simulink model "model1"  (R2020a)
settings: Solver=FixedStepAuto  StartTime=0.0  StopTime=30  FixedStep=0.005  RelTol=1e-3
values from neighbouring files (symbols this model uses):
  g = 9.81    [fast_init.m]
  I1 = 1    [fast_init.m]
  I2 = 10    [fast_init.m]
  ini_theta1 = 0    [fast_init.m]
  ini_theta1_d = 0    [fast_init.m]
  ini_theta2 = 0    [fast_init.m]
  ini_theta2_d = 0    [fast_init.m]
  ini_w = 1    [fast_init.m]
  ini_w_d = 0    [fast_init.m]
  ini_x0 = 0    [fast_init.m]
  ini_x0_d = 0    [fast_init.m]
  ini_x1 = ini_x0+r1*cos(pi/2 - ini_theta1)    [fast_init.m]
  ini_x1_d = 0    [fast_init.m]
  ini_x2 = ini_xH + r2*cos(pi/2 - ini_theta2)    [fast_init.m]
  ini_x2_d = 0    [fast_init.m]
  ini_y0 = 0.4    [fast_init.m]
  ini_y0_d = 0    [fast_init.m]
  ini_y1 = ini_y0+r1*sin(pi/2 - ini_theta1)    [fast_init.m]
  ini_y1_d = 0    [fast_init.m]
  ini_y2 = ini_yH + r2*sin(pi/2 - ini_theta2)    [fast_init.m]
  ini_y2_d = 0    [fast_init.m]
  M1 = 1    [fast_init.m]
  M2 = 10    [fast_init.m]
  r1 = 0.5    [fast_init.m]
  r2 = 0.4    [fast_init.m]
  theta1_des = 0    [fast_init.m]
libraries: cstblocks x6, simulink x1
settings Model: Creator=fabia  LastModifiedBy=mic-ciciolla

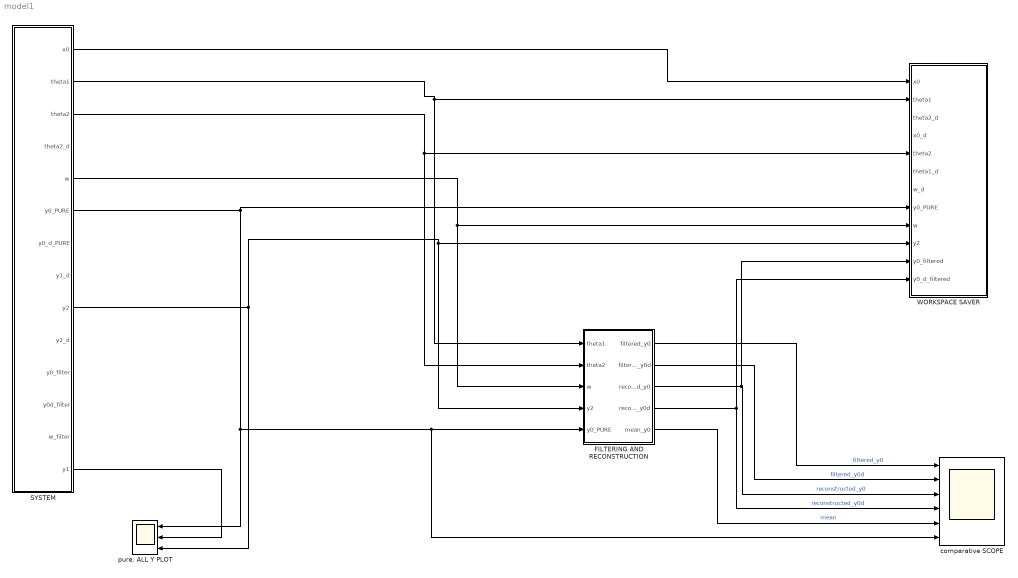
== system model1 ==
  FILTERING AND RECONSTRUCTION : Subsystem
  SYSTEM : Subsystem
  WORKSPACE SAVER : Subsystem
  comparative SCOPE : Scope  NumInputPorts=6
  pure: ALL Y PLOT : Scope  NumInputPorts=3
  wires:
  SYSTEM/6(y0_PURE) -> WORKSPACE SAVER/8(y0_PURE), pure: ALL Y PLOT/1, FILTERING AND RECONSTRUCTION/5(y0_PURE), comparative SCOPE/6
  SYSTEM/9(y2) -> FILTERING AND RECONSTRUCTION/4(y2), WORKSPACE SAVER/10(y2), pure: ALL Y PLOT/3
  SYSTEM/1(x0) -> WORKSPACE SAVER/1(x0)
  SYSTEM/2(theta1) -> FILTERING AND RECONSTRUCTION/1(theta1), WORKSPACE SAVER/2(theta1)
  SYSTEM/3(theta2) -> FILTERING AND RECONSTRUCTION/2(theta2), WORKSPACE SAVER/5(theta2)
  SYSTEM/5(w) -> FILTERING AND RECONSTRUCTION/3(w), WORKSPACE SAVER/9(w)
  SYSTEM/14(y1) -> pure: ALL Y PLOT/2
  FILTERING AND RECONSTRUCTION/1(filtered_y0) -> comparative SCOPE/1  "filtered_y0"
  FILTERING AND RECONSTRUCTION/2(filtered_y0d) -> comparative SCOPE/2  "filtered_y0d"
  FILTERING AND RECONSTRUCTION/4(reconstructed_y0d) -> WORKSPACE SAVER/12(y0_d_filtered), comparative SCOPE/4  "reconstructed_y0d"
  FILTERING AND RECONSTRUCTION/3(reconstructed_y0) -> WORKSPACE SAVER/11(y0_filtered), comparative SCOPE/3  "reconstructed_y0"
  FILTERING AND RECONSTRUCTION/5(mean_y0) -> comparative SCOPE/5  "mean"

== system model1/FILTERING AND RECONSTRUCTION ==
  theta1 : Inport
  theta2 : Inport  Port=2
  w : Inport  Port=3
  y2 : Inport  Port=4
  y0_PURE : Inport  Port=5
  FILTERING BLOCK : Subsystem
  RECONSTRUCTION BLOCK : Subsystem
  comparative SCOPE : Scope  NumInputPorts=5
  mean : MATLAB Function  TreatAsAtomicUnit=on
  filtered_y0 : Outport
  filtered_y0d : Outport  Port=2
  reconstructed_y0 : Outport  Port=3
  reconstructed_y0d : Outport  Port=4
  mean_y0 : Outport  Port=5
  wires:
  theta1/1 -> RECONSTRUCTION BLOCK/1(theta1)
  y0_PURE/1 -> FILTERING BLOCK/1(y0_PURE), comparative SCOPE/1
  y2/1 -> RECONSTRUCTION BLOCK/4(y2)
  theta2/1 -> RECONSTRUCTION BLOCK/2(theta2)
  RECONSTRUCTION BLOCK/1(reconstruct_y0) -> comparative SCOPE/2, mean/1(recon), reconstructed_y0/1
  FILTERING BLOCK/2(y0_d) -> filtered_y0d/1, comparative SCOPE/5  "filtered_y0d"
  RECONSTRUCTION BLOCK/2(recontruct_y0d) -> comparative SCOPE/3, reconstructed_y0d/1
  w/1 -> RECONSTRUCTION BLOCK/3(w)
  FILTERING BLOCK/1(y0) -> mean/2(filtered), filtered_y0/1, comparative SCOPE/4  "filtered_y0"
  mean/1(y) -> mean_y0/1

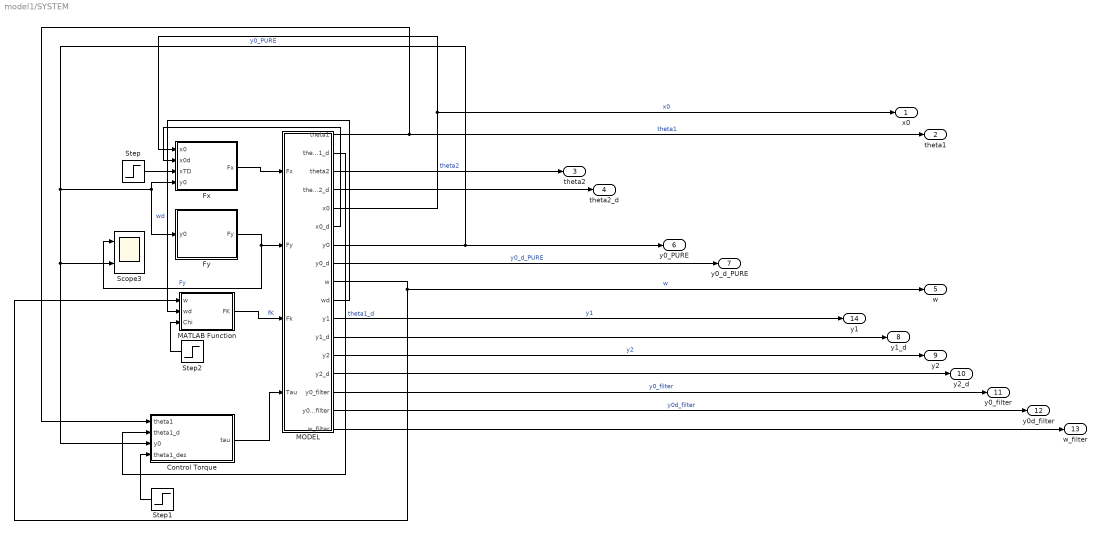
== system model1/SYSTEM ==
  Control Torque : MATLAB Function  TreatAsAtomicUnit=on
  Fx : MATLAB Function  TreatAsAtomicUnit=on
  Fy : MATLAB Function  TreatAsAtomicUnit=on
  MATLAB Function : MATLAB Function  TreatAsAtomicUnit=on
  MODEL : Subsystem
  Scope3 : Scope  NumInputPorts=2
  Step : Step  Time=0  After=0  SampleTime=0
  Step1 : Step  Time=0  After=theta1_des  SampleTime=0
  Step2 : Step  Time=0  After=0.0  SampleTime=0
  x0 : Outport
  theta1 : Outport  Port=2
  theta2 : Outport  Port=3
  theta2_d : Outport  Port=4
  w : Outport  Port=5
  y0_PURE : Outport  Port=6
  y0_d_PURE : Outport  Port=7
  y1_d : Outport  Port=8
  y2 : Outport  Port=9
  y2_d : Outport  Port=10
  y0_filter : Outport  Port=11
  y0d_filter : Outport  Port=12
  w_filter : Outport  Port=13
  y1 : Outport  Port=14
  wires:
  MODEL/2(theta1_d) -> Control Torque/2(theta1_d)  "theta1_d"
  MATLAB Function/1(FK) -> MODEL/3(Fk)  "fK"
  MODEL/9(w) -> w/1, MATLAB Function/1(w)  "w"
  MODEL/11(y1) -> y1/1  "y1"
  MODEL/14(y2_d) -> y2_d/1
  Fy/1(Fy) -> Scope3/1, MODEL/2(Fy)  "Fy"
  MODEL/17(w_filter) -> w_filter/1
  MODEL/12(y1_d) -> y1_d/1
  MODEL/5(x0) -> x0/1, Fx/1(x0)  "x0"
  MODEL/13(y2) -> y2/1  "y2"
  Fx/1(Fx) -> MODEL/1(Fx)
  MODEL/7(y0) -> y0_PURE/1, Control Torque/3(y0), Scope3/2, Fx/4(y0), Fy/1(y0)  "y0_PURE"
  MODEL/8(y0_d) -> y0_d_PURE/1  "y0_d_PURE"
  MODEL/1(theta1) -> Control Torque/1(theta1), theta1/1  "theta1"
  MODEL/15(y0_filter) -> y0_filter/1  "y0_filter"
  MODEL/3(theta2) -> theta2/1  "theta2"
  Step/1 -> Fx/3(xTD)
  MODEL/4(theta2_d) -> theta2_d/1
  MODEL/10(wd) -> MATLAB Function/2(wd)  "wd"
  MODEL/6(x0_d) -> Fx/2(x0d)
  MODEL/16("y0d_filter ") -> y0d_filter/1  "y0d_filter"
  Control Torque/1(tau) -> MODEL/4(Tau)
  Step1/1 -> Control Torque/4(theta1_des)
  Step2/1 -> MATLAB Function/3(Chi)

== system model1/WORKSPACE SAVER ==
  note: Workspace saver
  x0 : Inport
  theta1 : Inport  Port=2
  theta2_d : Inport  Port=3
  x0_d : Inport  Port=4
  theta2 : Inport  Port=5
  theta1_d : Inport  Port=6
  w_d : Inport  Port=7
  y0_PURE : Inport  Port=8
  w : Inport  Port=9
  y2 : Inport  Port=10
  y0_filtered : Inport  Port=11
  y0_d_filtered : Inport  Port=12
  "x : workspace state saver" : Subsystem
  "x_d : workspace state saver" : Subsystem
  wires:
  y0_PURE/1 -> "x : workspace state saver"/6(y0_pure)
  x0/1 -> "x : workspace state saver"/2(x0)
  theta1_d/1 -> "x_d : workspace state saver"/4(theta1_d)
  x0_d/1 -> "x_d : workspace state saver"/2(x0_d)
  w/1 -> "x : workspace state saver"/5(w)
  w_d/1 -> "x_d : workspace state saver"/5(w_d)
  y0_d_filtered/1 -> "x_d : workspace state saver"/3(y0_d)
  theta2_d/1 -> "x_d : workspace state saver"/1(theta2_d)
  theta2/1 -> "x : workspace state saver"/1(theta2)
  y2/1 -> "x : workspace state saver"/7(y2)
  y0_filtered/1 -> "x : workspace state saver"/3(y0)
  theta1/1 -> "x : workspace state saver"/4(theta1)

== system model1/FILTERING AND RECONSTRUCTION/FILTERING BLOCK ==
  note: derivaring&filtering the twice-filtered signal
  note: double filter on foot height
  note: comparing vel signals
  note: here i'm comparing height and vel signals
      | atm i'm considering good to choose the twice-filtered signals
  note: comparing y0 signals
  y0_PURE : Inport
  "Cut-Off Freq\t" : Constant  Value=45
  Cut-Off Freq2 : Constant  Value=53
  Derivative : Derivative
  FINAL SIGNALS test : Scope  NumInputPorts=2
  "HEIGHT : Comparing filters" : Scope  NumInputPorts=2
  RC LPF height : Subsystem
  "VERT_VEL :  Comparing filters" : Scope  NumInputPorts=2
  Varying LPF : cstblocks/Linear Parameter Varying/Varying Lowpass Filter  N=3
  Varying LPF2 : cstblocks/Linear Parameter Varying/Varying Lowpass Filter  N=2
  y0 : Outport
  y0_d : Outport  Port=2
  wires:
  Derivative/1 -> Varying LPF2/1  "y0_filtered_d_filtered_2"
  Varying LPF/1 -> FINAL SIGNALS test/1, y0/1, "HEIGHT : Comparing filters"/1, Derivative/1  "2_height_twice_filtered"
  "Cut-Off Freq\t"/1 -> Varying LPF/2
  Varying LPF2/1 -> FINAL SIGNALS test/2, y0_d/1, "VERT_VEL :  Comparing filters"/1  "2_vel_twice_filtered"
  Cut-Off Freq2/1 -> Varying LPF2/2
  y0_PURE/1 -> "HEIGHT : Comparing filters"/2, Varying LPF/1  "1_height_filter"

== system model1/FILTERING AND RECONSTRUCTION/RECONSTRUCTION BLOCK ==
  theta1 : Inport
  theta2 : Inport  Port=2
  w : Inport  Port=3
  y2 : Inport  Port=4
  Derivative : Derivative
  RECONSTRUCTION FUNCTION : MATLAB Function  TreatAsAtomicUnit=on
  reconstruct_y0 : Outport
  recontruct_y0d : Outport  Port=2
  wires:
  theta1/1 -> RECONSTRUCTION FUNCTION/3(theta1)
  w/1 -> RECONSTRUCTION FUNCTION/2(w)
  y2/1 -> RECONSTRUCTION FUNCTION/1(y2)
  RECONSTRUCTION FUNCTION/1(y0_r) -> reconstruct_y0/1, Derivative/1  "reconstruct_y0"
  theta2/1 -> RECONSTRUCTION FUNCTION/4(theta2)
  Derivative/1 -> recontruct_y0d/1  "recontruct_y0d"

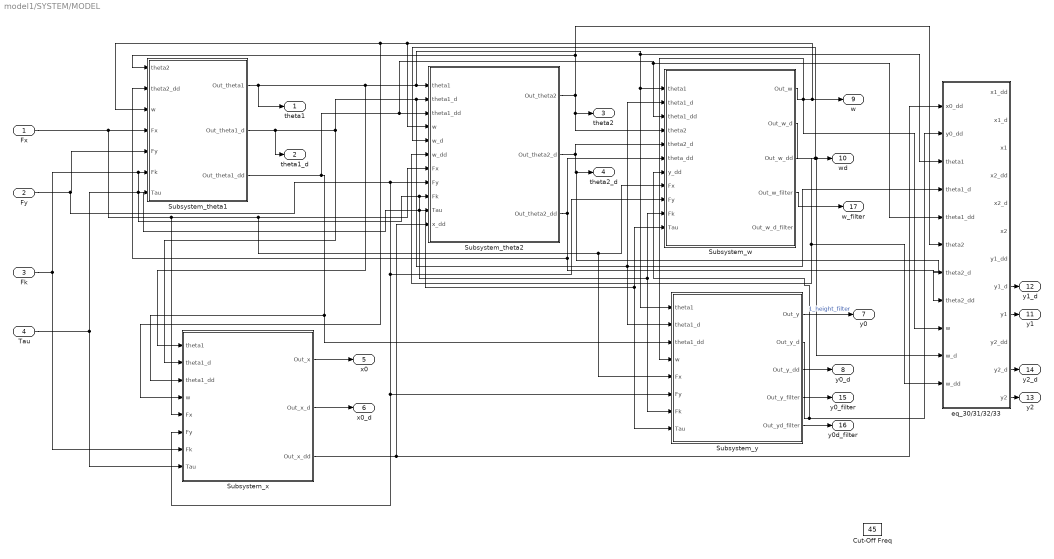
== system model1/SYSTEM/MODEL ==
  Fx : Inport
  Fy : Inport  Port=2
  Fk : Inport  Port=3
  Tau : Inport  Port=4
  "Cut-Off Freq\t" : Constant  Value=45
  Subsystem_theta1 : Subsystem
  Subsystem_theta2 : Subsystem
  Subsystem_w : Subsystem
  Subsystem_x : Subsystem
  Subsystem_y : Subsystem
  "eq_30/31/32/33 " : Subsystem
  theta1 : Outport
  theta1_d : Outport  Port=2
  theta2 : Outport  Port=3
  theta2_d : Outport  Port=4
  x0 : Outport  Port=5
  x0_d : Outport  Port=6
  y0 : Outport  Port=7
  y0_d : Outport  Port=8
  w : Outport  Port=9
  wd : Outport  Port=10
  y1 : Outport  Port=11
  y1_d : Outport  Port=12
  y2 : Outport  Port=13
  y2_d : Outport  Port=14
  y0_filter : Outport  Port=15
  "y0d_filter " : Outport  Port=16
  w_filter : Outport  Port=17
  wires:
  Subsystem_theta1/1(Out_theta1) -> Subsystem_x/1(theta1), "eq_30/31/32/33 "/3(theta1), Subsystem_y/1(theta1), Subsystem_w/1(theta1), Subsystem_theta2/1(theta1), theta1/1
  Subsystem_theta1/2(Out_theta1_d) -> Subsystem_y/2(theta1_d), "eq_30/31/32/33 "/4(theta1_d), Subsystem_w/2(theta1_d), Subsystem_theta2/2(theta1_d), Subsystem_x/2(theta1_d), theta1_d/1
  Subsystem_x/1(Out_x) -> x0/1
  Subsystem_x/2(Out_x_d) -> x0_d/1
  Subsystem_y/2(Out_y_d) -> y0_d/1
  "eq_30/31/32/33 "/9(y1) -> y1/1
  "eq_30/31/32/33 "/8(y1_d) -> y1_d/1
  "eq_30/31/32/33 "/12(y2) -> y2/1
  "eq_30/31/32/33 "/11(y2_d) -> y2_d/1
  Subsystem_w/2(Out_w_d) -> "eq_30/31/32/33 "/10(w_d), wd/1, Subsystem_theta2/5(w_d)
  Subsystem_w/1(Out_w) -> Subsystem_y/4(w), "eq_30/31/32/33 "/9(w), Subsystem_theta2/4(w), Subsystem_x/4(w), Subsystem_theta1/3(w), w/1
  Subsystem_theta2/1(Out_theta2) -> "eq_30/31/32/33 "/6(theta2), Subsystem_theta1/1(theta2), Subsystem_w/4(theta2), theta2/1
  Subsystem_theta2/2(Out_theta2_d) -> Subsystem_w/5(theta2_d), "eq_30/31/32/33 "/7(theta2_d), theta2_d/1
  Subsystem_theta1/3(Out_theta1_dd) -> Subsystem_x/3(theta1_dd), Subsystem_y/3(theta1_dd), "eq_30/31/32/33 "/5(theta1_dd), Subsystem_w/3(theta1_dd), Subsystem_theta2/3(theta1_dd)
  Subsystem_theta2/3(Out_theta2_dd) -> "eq_30/31/32/33 "/8(theta2_dd), Subsystem_theta1/2(theta2_dd), Subsystem_w/6(theta_dd)
  Subsystem_w/3(Out_w_dd) -> "eq_30/31/32/33 "/11(w_dd), Subsystem_theta2/6(w_dd)
  Subsystem_y/3(Out_y_dd) -> "eq_30/31/32/33 "/2(y0_dd), Subsystem_w/7(y_dd)
  Subsystem_x/3(Out_x_dd) -> "eq_30/31/32/33 "/1(x0_dd), Subsystem_theta2/11(x_dd)
  Fx/1 -> Subsystem_x/5(Fx), Subsystem_y/5(Fx), Subsystem_w/8(Fx), Subsystem_theta2/7(Fx), Subsystem_theta1/4(Fx)
  Fy/1 -> Subsystem_w/9(Fy), Subsystem_x/6(Fy), Subsystem_y/6(Fy), Subsystem_theta2/8(Fy), Subsystem_theta1/5(Fy)
  Fk/1 -> Subsystem_x/7(Fk), Subsystem_y/7(Fk), Subsystem_w/10(Fk), Subsystem_theta2/9(Fk), Subsystem_theta1/6(Fk)
  Tau/1 -> Subsystem_x/8(Tau), Subsystem_y/8(Tau), Subsystem_w/11(Tau), Subsystem_theta2/10(Tau), Subsystem_theta1/7(Tau)
  Subsystem_y/4(Out_y_filter) -> y0_filter/1
  Subsystem_y/5(Out_yd_filter) -> "y0d_filter "/1
  Subsystem_y/1(Out_y) -> y0/1  "1_height_filter"
  Subsystem_w/4(Out_w_filter) -> w_filter/1

== system model1/WORKSPACE SAVER/x : workspace state saver ==
  theta2 : Inport
  x0 : Inport  Port=2
  y0 : Inport  Port=3
  theta1 : Inport  Port=4
  w : Inport  Port=5
  y0_pure : Inport  Port=6
  y2 : Inport  Port=7
  state: theta1 : ToWorkspace  VariableName=theta1  SampleTime=-1
  state: theta2 : ToWorkspace  VariableName=theta2  SaveFormat=Structure With Time  SampleTime=-1
  state: w : ToWorkspace  VariableName=lenght  SampleTime=-1
  state: x : ToWorkspace  VariableName=horizontal  SampleTime=-1
  "state: y " : ToWorkspace  VariableName=height  SampleTime=-1
  state: y0_pure : ToWorkspace  VariableName=y0_pure  SampleTime=-1
  state: y2 : ToWorkspace  VariableName=y2  SampleTime=-1
  wires:
  w/1 -> state: w/1
  theta2/1 -> state: theta2/1
  theta1/1 -> state: theta1/1
  x0/1 -> state: x/1
  y0/1 -> "state: y "/1
  y0_pure/1 -> state: y0_pure/1
  y2/1 -> state: y2/1

== system model1/WORKSPACE SAVER/x_d : workspace state saver ==
  theta2_d : Inport
  x0_d : Inport  Port=2
  y0_d : Inport  Port=3
  theta1_d : Inport  Port=4
  w_d : Inport  Port=5
  state: theta1_d : ToWorkspace  VariableName=theta1_d  SampleTime=-1
  state: theta2_d : ToWorkspace  VariableName=theta2_d  SaveFormat=Structure  SampleTime=-1
  state: w_d : ToWorkspace  VariableName=lenght_d  SampleTime=-1
  state: x_d : ToWorkspace  VariableName=horizontal_d  SampleTime=-1
  "state: y_d " : ToWorkspace  VariableName=height_d  SampleTime=-1
  wires:
  w_d/1 -> state: w_d/1
  theta2_d/1 -> state: theta2_d/1
  theta1_d/1 -> state: theta1_d/1
  x0_d/1 -> state: x_d/1
  y0_d/1 -> "state: y_d "/1

== system model1/FILTERING AND RECONSTRUCTION/FILTERING BLOCK/RC LPF height ==
  In1 : Inport
  Add : Sum  Inputs=+-
  Discrete Derivative : simulink/Discrete/Discrete Derivative  gainval=0.055  ICPrevScaledInput=ini_y0  OutMin=[]  OutMax=[]  OutDataType=fixdt(1, 16)  OutScaling=2^-10  DoSatur=off
  Out1 : Outport
  wires:
  In1/1 -> Add/1
  Add/1 -> Discrete Derivative/1, Out1/1
  Discrete Derivative/1 -> Add/2

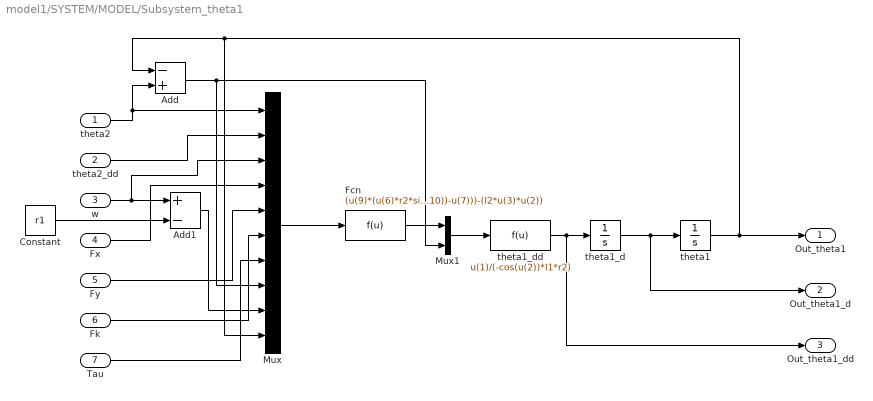
== system model1/SYSTEM/MODEL/Subsystem_theta1 ==
  theta2 : Inport
  theta2_dd : Inport  Port=2
  w : Inport  Port=3
  Fx : Inport  Port=4
  Fy : Inport  Port=5
  Fk : Inport  Port=6
  Tau : Inport  Port=7
  Add : Sum  Inputs=-+
  Add1 : Sum  Inputs=+-
  Constant : Constant  Value=r1
  Fcn : Fcn  Expr=(u(9)*(u(6)*r2*sin(u(8))+u(7)))-(r2*cos(u(8))*(r1*u(5)*sin(u(10))-r1*u(4)*cos(u(10))-u(7)))-(I2*u(3)*u(2))
  Mux : Mux  Inputs=10
  Mux1 : Mux  Inputs=2
  theta1 : Integrator  InitialCondition=ini_theta1  LimitOutput=on  UpperSaturationLimit=pi/2  LowerSaturationLimit=-pi/2
  theta1_d : Integrator  InitialCondition=ini_theta1_d  LimitOutput=on  UpperSaturationLimit=pi/2  LowerSaturationLimit=-pi/2
  theta1_dd : Fcn  Expr=u(1)/(-cos(u(2))*I1*r2)
  Out_theta1 : Outport
  Out_theta1_d : Outport  Port=2
  Out_theta1_dd : Outport  Port=3
  wires:
  theta2/1 -> Mux/1, Add/2
  theta1/1 -> Out_theta1/1, Mux/10, Add/1
  w/1 -> Mux/3, Add1/1
  Constant/1 -> Add1/2
  theta2_dd/1 -> Mux/2
  Fx/1 -> Mux/4
  Fy/1 -> Mux/5
  Fk/1 -> Mux/6
  Tau/1 -> Mux/7
  Add/1 -> Mux/8, Mux1/2
  Add1/1 -> Mux/9
  Mux/1 -> Fcn/1
  Fcn/1 -> Mux1/1
  Mux1/1 -> theta1_dd/1
  theta1_dd/1 -> Out_theta1_dd/1, theta1_d/1
  theta1_d/1 -> Out_theta1_d/1, theta1/1

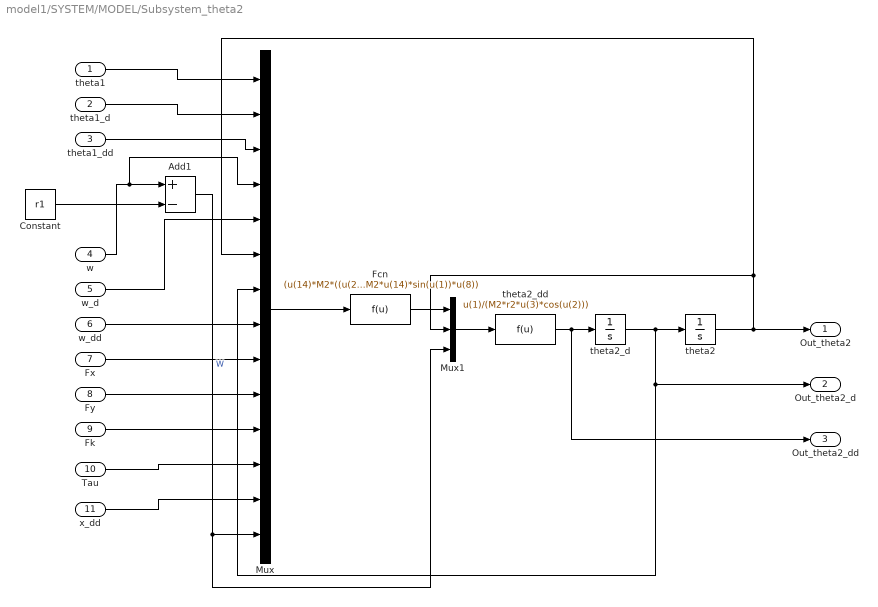
== system model1/SYSTEM/MODEL/Subsystem_theta2 ==
  theta1 : Inport
  theta1_d : Inport  Port=2
  theta1_dd : Inport  Port=3
  w : Inport  Port=4
  w_d : Inport  Port=5
  w_dd : Inport  Port=6
  Fx : Inport  Port=7
  Fy : Inport  Port=8
  Fk : Inport  Port=9
  Tau : Inport  Port=10
  x_dd : Inport  Port=11
  Add1 : Sum  Inputs=+-
  Constant : Constant  Value=r1
  Fcn : Fcn  Expr=(u(14)*M2*((u(2)^2)*u(14)*sin(u(1))-2*u(2)*u(5)*cos(u(1))+r2*(u(7)^2)*sin(u(6))+r1*(u(2)^2)*sin(u(1))))-(r1*u(9)*(cos(u(1)))^2)+(cos(u(1))*(r1*u(10)*sin(u(1))-u(12)))+(u(11)*u(14)*sin(u(1)))-(M2*u(14)*u(13))-(cos(u(1))*(M2*u(14)*u(4)+I1)*u(3))-(M2*u(14)*sin(u(1))*u(8))
  Mux : Mux  Inputs=14
  Mux1 : Mux  Inputs=3
  theta2 : Integrator  InitialCondition=ini_theta2
  theta2_d : Integrator  InitialCondition=ini_theta2_d
  theta2_dd : Fcn  Expr=u(1)/(M2*r2*u(3)*cos(u(2)))
  Out_theta2 : Outport
  Out_theta2_d : Outport  Port=2
  Out_theta2_dd : Outport  Port=3
  wires:
  theta2/1 -> Mux1/2, Mux/6, Out_theta2/1
  Fcn/1 -> Mux1/1
  Mux1/1 -> theta2_dd/1
  theta2_dd/1 -> Out_theta2_dd/1, theta2_d/1
  theta2_d/1 -> Mux/7, Out_theta2_d/1, theta2/1
  Constant/1 -> Add1/2
  theta1/1 -> Mux/1
  theta1_d/1 -> Mux/2
  theta1_dd/1 -> Mux/3
  Add1/1 -> Mux1/3, Mux/14  "W"
  Mux/1 -> Fcn/1
  w/1 -> Mux/4, Add1/1
  w_d/1 -> Mux/5
  w_dd/1 -> Mux/8
  Fx/1 -> Mux/9
  Fy/1 -> Mux/10
  Fk/1 -> Mux/11
  Tau/1 -> Mux/12
  x_dd/1 -> Mux/13

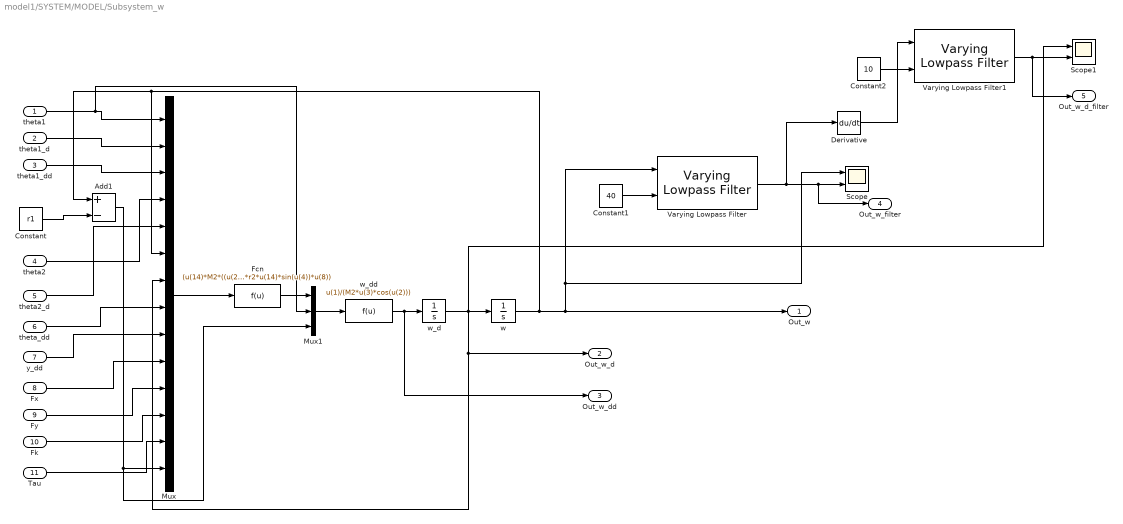
== system model1/SYSTEM/MODEL/Subsystem_w ==
  theta1 : Inport
  theta1_d : Inport  Port=2
  theta1_dd : Inport  Port=3
  theta2 : Inport  Port=4
  theta2_d : Inport  Port=5
  theta_dd : Inport  Port=6
  y_dd : Inport  Port=7
  Fx : Inport  Port=8
  Fy : Inport  Port=9
  Fk : Inport  Port=10
  Tau : Inport  Port=11
  Add1 : Sum  Inputs=+-
  Constant : Constant  Value=r1
  Constant1 : Constant  Value=40
  Constant2 : Constant  Value=10
  Derivative : Derivative
  Fcn : Fcn  Expr=(u(14)*M2*((u(2)^2)*u(14)*cos(u(1))+2*u(2)*u(7)*sin(u(1))+r2*(u(5)^2)*cos(u(4))+r1*(u(2)^2)*cos(u(1))-g))+(r1*u(10)*cos(u(1))*sin(u(1)))-(sin(u(1))*(r1*u(11)*sin(u(1))-u(13)))+(u(12)*u(14)*cos(u(1)))+(sin(u(1))*(M2*u(14)*u(6)+I1)*u(3))-(M2*u(14)*u(9))+(M2*r2*u(14)*sin(u(4))*u(8))
  Mux : Mux  Inputs=14
  Mux1 : Mux  Inputs=3
  Scope : Scope  NumInputPorts=2
  Scope1 : Scope  NumInputPorts=2
  Varying Lowpass Filter : cstblocks/Linear Parameter Varying/Varying Lowpass Filter  N=1
  Varying Lowpass Filter1 : cstblocks/Linear Parameter Varying/Varying Lowpass Filter  N=1
  w : Integrator  InitialCondition=ini_w
  w_d : Integrator  InitialCondition=ini_w_d
  w_dd : Fcn  Expr=u(1)/(M2*u(3)*cos(u(2)))
  Out_w : Outport
  Out_w_d : Outport  Port=2
  Out_w_dd : Outport  Port=3
  Out_w_filter : Outport  Port=4
  Out_w_d_filter : Outport  Port=5
  wires:
  Fcn/1 -> Mux1/1
  Mux1/1 -> w_dd/1
  w_dd/1 -> Out_w_dd/1, w_d/1
  w_d/1 -> Scope1/1, Mux/7, Out_w_d/1, w/1
  Constant/1 -> Add1/2
  Mux/1 -> Fcn/1
  Add1/1 -> Mux1/3, Mux/14
  theta1/1 -> Mux1/2, Mux/1
  theta1_d/1 -> Mux/2
  theta1_dd/1 -> Mux/3
  theta2/1 -> Mux/4
  theta2_d/1 -> Mux/5
  theta_dd/1 -> Mux/8
  y_dd/1 -> Mux/9
  Fx/1 -> Mux/10
  Fy/1 -> Mux/11
  Fk/1 -> Mux/12
  Tau/1 -> Mux/13
  Constant1/1 -> Varying Lowpass Filter/2
  w/1 -> Mux/6, Add1/1, Out_w/1, Scope/1, Varying Lowpass Filter/1
  Derivative/1 -> Varying Lowpass Filter1/1
  Constant2/1 -> Varying Lowpass Filter1/2
  Varying Lowpass Filter/1 -> Derivative/1, Out_w_filter/1, Scope/2
  Varying Lowpass Filter1/1 -> Out_w_d_filter/1, Scope1/2

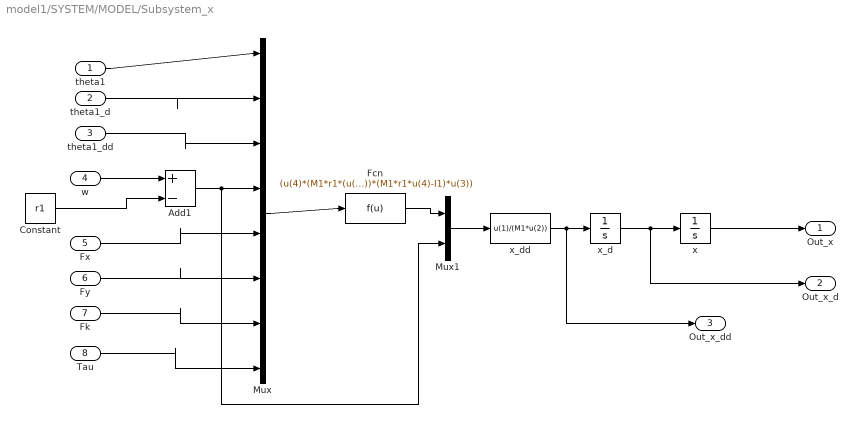
== system model1/SYSTEM/MODEL/Subsystem_x ==
  theta1 : Inport
  theta1_d : Inport  Port=2
  theta1_dd : Inport  Port=3
  w : Inport  Port=4
  Fx : Inport  Port=5
  Fy : Inport  Port=6
  Fk : Inport  Port=7
  Tau : Inport  Port=8
  Add1 : Sum  Inputs=+-
  Constant : Constant  Value=r1
  Fcn : Fcn  Expr=(u(4)*(M1*r1*(u(2)^2)*sin(u(1))-u(7)*sin(u(1))+u(5)))-(cos(u(1))*(u(6)*r1*sin(u(1))-u(5)*r1*cos(u(1))-u(8)))-(cos(u(1))*(M1*r1*u(4)-I1)*u(3))
  Mux : Mux  Inputs=8
  Mux1 : Mux  Inputs=2
  x : Integrator  InitialCondition=ini_x0
  x_d : Integrator  InitialCondition=ini_x0_d
  x_dd : Fcn  Expr=u(1)/(M1*u(2))
  Out_x : Outport
  Out_x_d : Outport  Port=2
  Out_x_dd : Outport  Port=3
  wires:
  x/1 -> Out_x/1
  Fcn/1 -> Mux1/1
  Mux1/1 -> x_dd/1
  x_dd/1 -> Out_x_dd/1, x_d/1
  x_d/1 -> Out_x_d/1, x/1
  Constant/1 -> Add1/2
  Mux/1 -> Fcn/1
  w/1 -> Add1/1
  theta1/1 -> Mux/1
  theta1_d/1 -> Mux/2
  theta1_dd/1 -> Mux/3
  Add1/1 -> Mux1/2, Mux/4
  Fx/1 -> Mux/5
  Fy/1 -> Mux/6
  Fk/1 -> Mux/7
  Tau/1 -> Mux/8

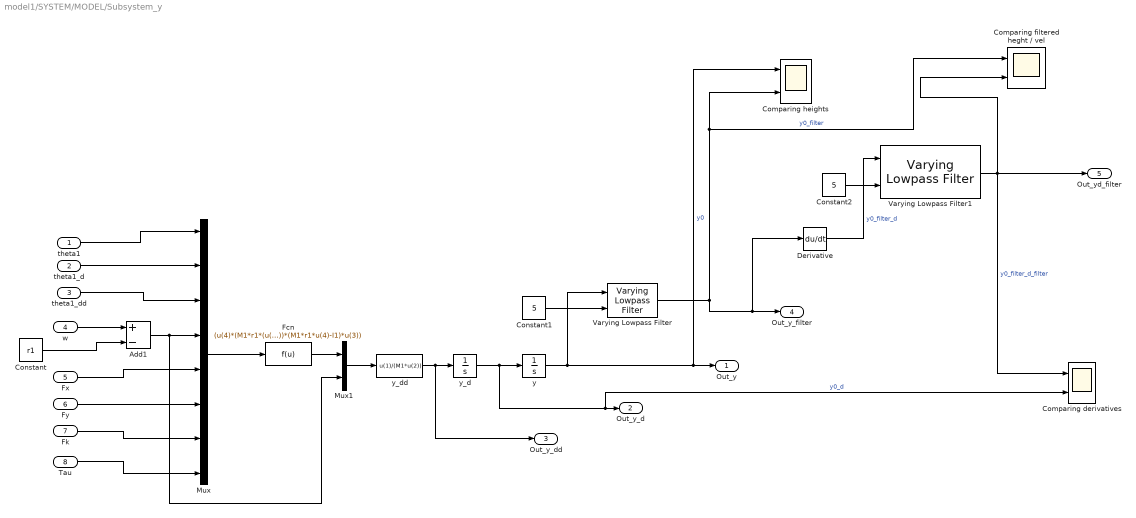
== system model1/SYSTEM/MODEL/Subsystem_y ==
  theta1 : Inport
  theta1_d : Inport  Port=2
  theta1_dd : Inport  Port=3
  w : Inport  Port=4
  Fx : Inport  Port=5
  Fy : Inport  Port=6
  Fk : Inport  Port=7
  Tau : Inport  Port=8
  Add1 : Sum  Inputs=+-
  Comparing derivatives : Scope  NumInputPorts=2
  Comparing filtered heght / vel : Scope  NumInputPorts=2
  Comparing heights : Scope  NumInputPorts=2
  Constant : Constant  Value=r1
  Constant1 : Constant  Value=5
  Constant2 : Constant  Value=5
  Derivative : Derivative
  Fcn : Fcn  Expr=(u(4)*(M1*r1*(u(2)^2)*cos(u(1))-u(7)*cos(u(1))+u(6)-M1*g))-(sin(u(1))*(u(6)*r1*sin(u(1))-u(5)*r1*cos(u(1))-u(8)))+(sin(u(1))*(M1*r1*u(4)-I1)*u(3))
  Mux : Mux  Inputs=8
  Mux1 : Mux  Inputs=2
  Varying Lowpass Filter : cstblocks/Linear Parameter Varying/Varying Lowpass Filter  N=1
  Varying Lowpass Filter1 : cstblocks/Linear Parameter Varying/Varying Lowpass Filter  N=1
  y : Integrator  InitialCondition=ini_y0
  y_d : Integrator  InitialCondition=ini_y0_d
  y_dd : Fcn  Expr=u(1)/(M1*u(2))
  Out_y : Outport
  Out_y_d : Outport  Port=2
  Out_y_dd : Outport  Port=3
  Out_y_filter : Outport  Port=4
  Out_yd_filter : Outport  Port=5
  wires:
  Fcn/1 -> Mux1/1
  Mux1/1 -> y_dd/1
  y_dd/1 -> Out_y_dd/1, y_d/1
  y_d/1 -> Comparing derivatives/2, Out_y_d/1, y/1  "y0_d"
  Constant/1 -> Add1/2
  Mux/1 -> Fcn/1
  w/1 -> Add1/1
  theta1/1 -> Mux/1
  theta1_d/1 -> Mux/2
  theta1_dd/1 -> Mux/3
  Add1/1 -> Mux1/2, Mux/4
  Fx/1 -> Mux/5
  Fy/1 -> Mux/6
  Fk/1 -> Mux/7
  Tau/1 -> Mux/8
  Constant1/1 -> Varying Lowpass Filter/2
  Varying Lowpass Filter/1 -> Comparing filtered heght / vel/1, Comparing heights/2, Derivative/1, Out_y_filter/1  "y0_filter"
  Constant2/1 -> Varying Lowpass Filter1/2
  Derivative/1 -> Varying Lowpass Filter1/1  "y0_filter_d"
  Varying Lowpass Filter1/1 -> Comparing filtered heght / vel/2, Comparing derivatives/1, Out_yd_filter/1  "y0_filter_d_filter"
  y/1 -> Comparing heights/1, Out_y/1, Varying Lowpass Filter/1  "y0"

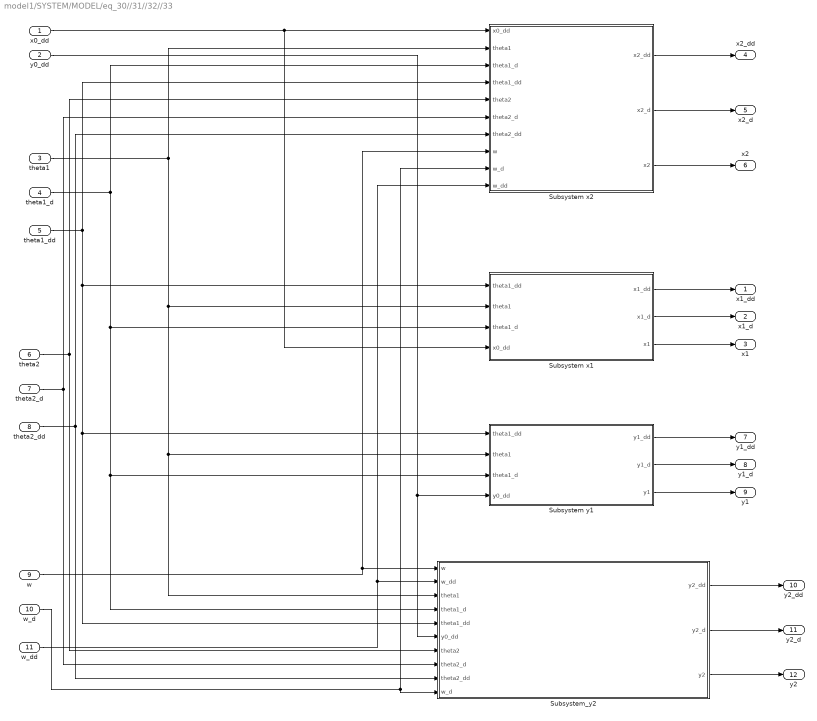
== system model1/SYSTEM/MODEL/eq_30//31//32//33  ==
  x0_dd : Inport
  y0_dd : Inport  Port=2
  theta1 : Inport  Port=3
  theta1_d : Inport  Port=4
  theta1_dd : Inport  Port=5
  theta2 : Inport  Port=6
  theta2_d : Inport  Port=7
  theta2_dd : Inport  Port=8
  w : Inport  Port=9
  w_d : Inport  Port=10
  w_dd : Inport  Port=11
  Subsystem x1 : Subsystem
  Subsystem x2 : Subsystem
  Subsystem y1 : Subsystem
  Subsystem_y2 : Subsystem
  x1_dd : Outport
  x1_d : Outport  Port=2
  x1 : Outport  Port=3
  x2_dd : Outport  Port=4
  x2_d : Outport  Port=5
  x2 : Outport  Port=6
  y1_dd : Outport  Port=7
  y1_d : Outport  Port=8
  y1 : Outport  Port=9
  y2_dd : Outport  Port=10
  y2_d : Outport  Port=11
  y2 : Outport  Port=12
  wires:
  Subsystem x1/1(x1_dd) -> x1_dd/1
  Subsystem x1/3(x1) -> x1/1
  x0_dd/1 -> Subsystem x1/4(x0_dd), Subsystem x2/1(x0_dd)
  Subsystem_y2/1(y2_dd) -> y2_dd/1
  theta1_d/1 -> Subsystem_y2/4(theta1_d), Subsystem y1/3(theta1_d), Subsystem x1/3(theta1_d), Subsystem x2/3(theta1_d)
  Subsystem x2/1(x2_dd) -> x2_dd/1
  Subsystem x2/3(x2) -> x2/1
  w_dd/1 -> Subsystem x2/10(w_dd), Subsystem_y2/2(w_dd)
  Subsystem_y2/3(y2) -> y2/1
  theta1/1 -> Subsystem_y2/3(theta1), Subsystem y1/2(theta1), Subsystem x1/2(theta1), Subsystem x2/2(theta1)
  Subsystem x1/2(x1_d) -> x1_d/1
  theta1_dd/1 -> Subsystem_y2/5(theta1_dd), Subsystem y1/1("theta1_dd "), Subsystem x1/1("theta1_dd "), Subsystem x2/4(theta1_dd)
  y0_dd/1 -> Subsystem_y2/6(y0_dd), Subsystem y1/4(y0_dd)
  theta2_dd/1 -> Subsystem x2/7("theta2_dd "), Subsystem_y2/9(theta2_dd)
  w_d/1 -> Subsystem_y2/10(w_d), Subsystem x2/9(w_d)
  Subsystem x2/2(x2_d) -> x2_d/1
  Subsystem y1/3(y1) -> y1/1
  theta2_d/1 -> Subsystem x2/6(theta2_d), Subsystem_y2/8(theta2_d)
  theta2/1 -> Subsystem x2/5(theta2), Subsystem_y2/7(theta2)
  w/1 -> Subsystem x2/8(w), Subsystem_y2/1(w)
  Subsystem y1/2(y1_d) -> y1_d/1
  Subsystem y1/1(y1_dd) -> y1_dd/1
  Subsystem_y2/2(y2_d) -> y2_d/1

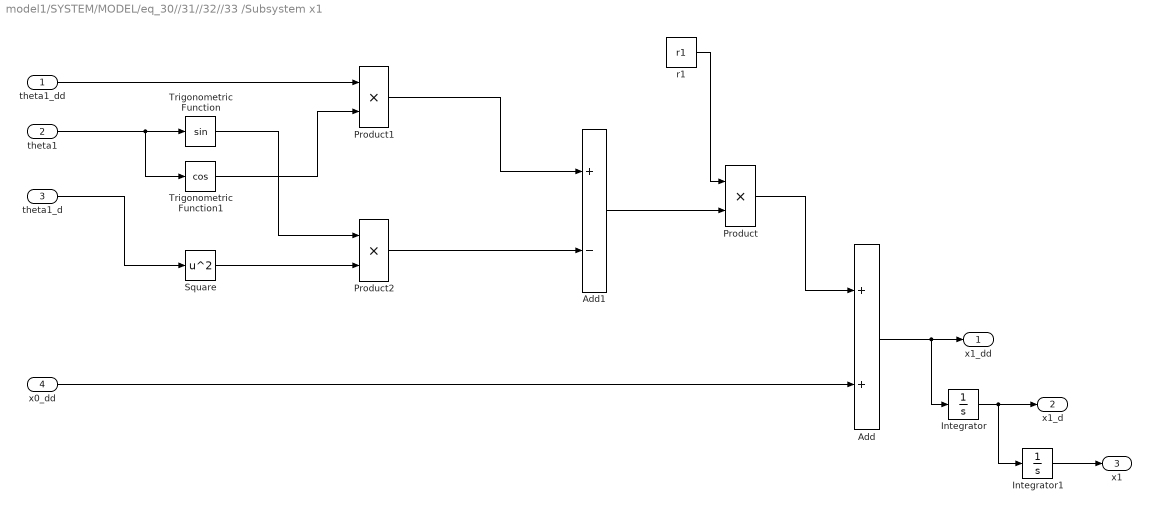
== system model1/SYSTEM/MODEL/eq_30//31//32//33 /Subsystem x1 ==
  "theta1_dd " : Inport
  theta1 : Inport  Port=2
  theta1_d : Inport  Port=3
  x0_dd : Inport  Port=4
  Add : Sum
  Add1 : Sum  Inputs=+-
  Integrator : Integrator  InitialCondition=ini_x1_d
  Integrator1 : Integrator  InitialCondition=ini_x1
  Product : Product
  Product1 : Product
  Product2 : Product
  Square : Math  Operator=square  SaturateOnIntegerOverflow=on
  Trigonometric Function : Trigonometry
  Trigonometric Function1 : Trigonometry  Operator=cos
  r1 : Constant  Value=r1
  x1_dd : Outport
  x1_d : Outport  Port=2
  x1 : Outport  Port=3
  wires:
  Add1/1 -> Product/2
  Product/1 -> Add/1
  Product2/1 -> Add1/2
  r1/1 -> Product/1
  Trigonometric Function1/1 -> Product1/2
  x0_dd/1 -> Add/2
  theta1_d/1 -> Square/1
  Trigonometric Function/1 -> Product2/1
  Integrator/1 -> x1_d/1, Integrator1/1
  Add/1 -> x1_dd/1, Integrator/1
  Square/1 -> Product2/2
  Product1/1 -> Add1/1
  "theta1_dd "/1 -> Product1/1
  theta1/1 -> Trigonometric Function1/1, Trigonometric Function/1
  Integrator1/1 -> x1/1

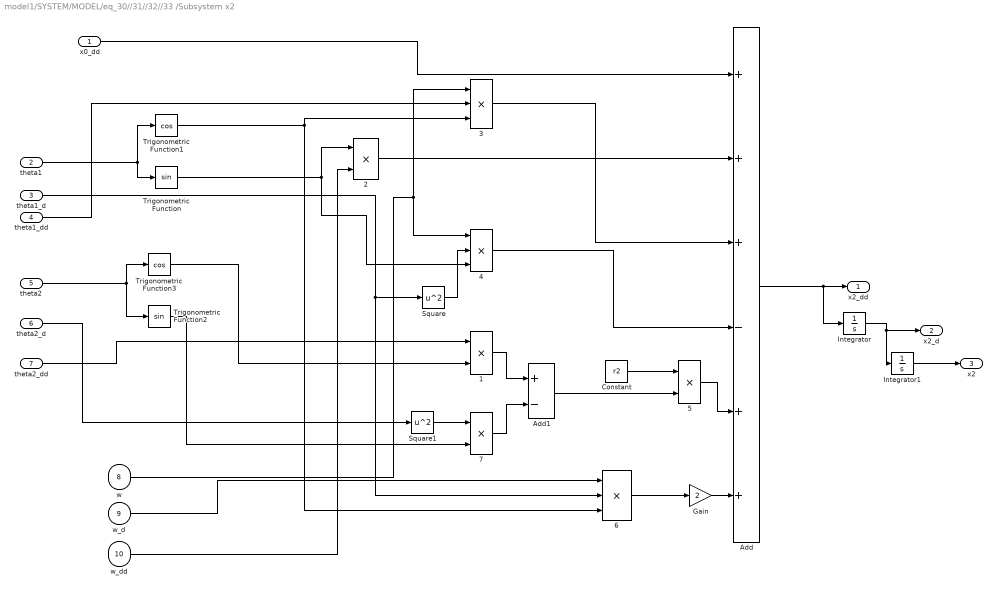
== system model1/SYSTEM/MODEL/eq_30//31//32//33 /Subsystem x2 ==
  x0_dd : Inport
  theta1 : Inport  Port=2
  theta1_d : Inport  Port=3
  theta1_dd : Inport  Port=4
  theta2 : Inport  Port=5
  theta2_d : Inport  Port=6
  "theta2_dd " : Inport  Port=7
  w : Inport  Port=8
  w_d : Inport  Port=9
  w_dd : Inport  Port=10
  {1..2,5,7} (4 alike) : Product
  3 : Product  Inputs=3
  4 : Product  Inputs=3
  6 : Product  Inputs=3
  Add : Sum  Inputs=+++-++
  Add1 : Sum  Inputs=+-
  Constant : Constant  Value=r2
  Gain : Gain  Gain=2
  Integrator : Integrator  InitialCondition=ini_x2_d
  Integrator1 : Integrator  InitialCondition=ini_x2
  Square : Math  Operator=square  SaturateOnIntegerOverflow=on
  Square1 : Math  Operator=square  SaturateOnIntegerOverflow=on
  Trigonometric Function : Trigonometry
  Trigonometric Function1 : Trigonometry  Operator=cos
  Trigonometric Function2 : Trigonometry
  Trigonometric Function3 : Trigonometry  Operator=cos
  x2_dd : Outport
  x2_d : Outport  Port=2
  x2 : Outport  Port=3
  wires:
  7/1 -> Add1/2
  Integrator1/1 -> x2/1
  w_d/1 -> 6/1
  Constant/1 -> 5/1
  Integrator/1 -> x2_d/1, Integrator1/1
  Trigonometric Function1/1 -> 6/3, 3/3
  x0_dd/1 -> Add/1
  Add1/1 -> 5/2
  theta2/1 -> Trigonometric Function3/1, Trigonometric Function2/1
  6/1 -> Gain/1
  4/1 -> Add/4
  Square/1 -> 4/2
  theta1_d/1 -> 6/2, Square/1
  Square1/1 -> 7/1
  w/1 -> 3/1, 4/1
  Add/1 -> x2_dd/1, Integrator/1
  Trigonometric Function2/1 -> 7/2
  Trigonometric Function3/1 -> 1/2
  w_dd/1 -> 2/2
  theta1/1 -> Trigonometric Function1/1, Trigonometric Function/1
  Gain/1 -> Add/6
  Trigonometric Function/1 -> 4/3, 2/1
  theta1_dd/1 -> 3/2
  3/1 -> Add/3
  1/1 -> Add1/1
  2/1 -> Add/2
  5/1 -> Add/5
  "theta2_dd "/1 -> 1/1
  theta2_d/1 -> Square1/1

== system model1/SYSTEM/MODEL/eq_30//31//32//33 /Subsystem y1 ==
  "theta1_dd " : Inport
  theta1 : Inport  Port=2
  theta1_d : Inport  Port=3
  y0_dd : Inport  Port=4
  Add : Sum  Inputs=-+
  Add1 : Sum
  Integrator : Integrator  InitialCondition=ini_y1_d
  Integrator1 : Integrator  InitialCondition=ini_y1
  Product : Product
  Product1 : Product
  Product2 : Product
  Square : Math  Operator=square  SaturateOnIntegerOverflow=on
  Trigonometric Function : Trigonometry
  Trigonometric Function1 : Trigonometry  Operator=cos
  r1 : Constant  Value=r1
  y1_dd : Outport
  y1_d : Outport  Port=2
  y1 : Outport  Port=3
  wires:
  "theta1_dd "/1 -> Product1/1
  Product1/1 -> Add1/1
  y0_dd/1 -> Add/2
  Integrator/1 -> y1_d/1, Integrator1/1
  Add/1 -> y1_dd/1, Integrator/1
  r1/1 -> Product/1
  Integrator1/1 -> y1/1
  theta1/1 -> Trigonometric Function1/1, Trigonometric Function/1
  Square/1 -> Product2/2
  theta1_d/1 -> Square/1
  Product/1 -> Add/1
  Trigonometric Function/1 -> Product1/2
  Product2/1 -> Add1/2
  Add1/1 -> Product/2
  Trigonometric Function1/1 -> Product2/1

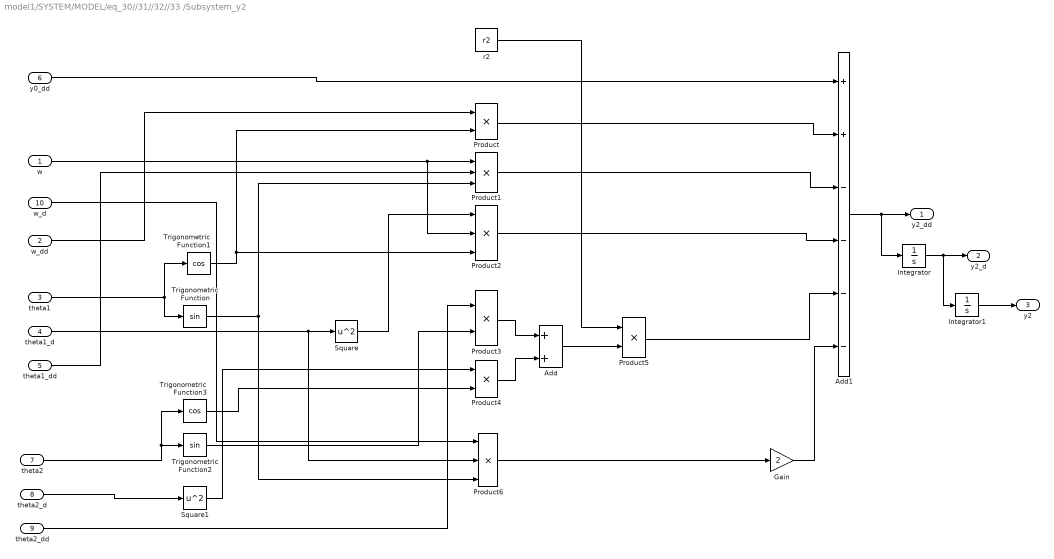
== system model1/SYSTEM/MODEL/eq_30//31//32//33 /Subsystem_y2 ==
  w : Inport
  w_dd : Inport  Port=2
  theta1 : Inport  Port=3
  theta1_d : Inport  Port=4
  theta1_dd : Inport  Port=5
  y0_dd : Inport  Port=6
  theta2 : Inport  Port=7
  theta2_d : Inport  Port=8
  theta2_dd : Inport  Port=9
  w_d : Inport  Port=10
  Add : Sum
  Add1 : Sum  Inputs=++----
  Gain : Gain  Gain=2
  Integrator : Integrator  InitialCondition=ini_y2_d
  Integrator1 : Integrator  InitialCondition=ini_y2
  Product{,3..5} (4 alike) : Product
  Product1 : Product  Inputs=3
  Product2 : Product  Inputs=3
  Product6 : Product  Inputs=3
  Square : Math  Operator=square  SaturateOnIntegerOverflow=on
  Square1 : Math  Operator=square  SaturateOnIntegerOverflow=on
  Trigonometric Function : Trigonometry
  Trigonometric Function1 : Trigonometry  Operator=cos
  Trigonometric Function2 : Trigonometry
  Trigonometric Function3 : Trigonometry  Operator=cos
  r2 : Constant  Value=r2
  y2_dd : Outport
  y2_d : Outport  Port=2
  y2 : Outport  Port=3
  wires:
  r2/1 -> Product5/1
  Product2/1 -> Add1/4
  theta2_d/1 -> Square1/1
  Product5/1 -> Add1/5
  Product1/1 -> Add1/3
  y0_dd/1 -> Add1/1
  Product3/1 -> Add/1
  Product6/1 -> Gain/1
  theta1_d/1 -> Product6/2, Square/1
  Integrator1/1 -> y2/1
  w/1 -> Product2/2, Product1/1
  Trigonometric Function/1 -> Product1/3, Product6/3
  theta1_dd/1 -> Product1/2
  Integrator/1 -> y2_d/1, Integrator1/1
  Product/1 -> Add1/2
  w_d/1 -> Product6/1
  theta1/1 -> Trigonometric Function1/1, Trigonometric Function/1
  w_dd/1 -> Product/1
  Gain/1 -> Add1/6
  Trigonometric Function1/1 -> Product/2, Product2/3
  Square1/1 -> Product4/1
  theta2/1 -> Trigonometric Function3/1, Trigonometric Function2/1
  Add1/1 -> y2_dd/1, Integrator/1
  Product4/1 -> Add/2
  Trigonometric Function2/1 -> Product3/2
  Trigonometric Function3/1 -> Product4/2
  Add/1 -> Product5/2
  Square/1 -> Product2/1
  theta2_dd/1 -> Product3/1

== matlab function model1/SYSTEM/Fx ==
  data: x0 input; Fx output; x0d input; xTD input; y0 input
function Fx = fcn(x0,x0d,xTD,y0)
KG=10^4; % [Nt/m]
BG=75; % [Nt-s/m]
if y0<0
   Fx = -KG*(x0-xTD)-(BG*x0d);
else
   Fx=0;
end

== matlab function model1/SYSTEM/Fy ==
  data: Fy output; y0 input
function Fy = fcn(y0)
KG=10^4; % [Nt/m]
BG=75; % [Nt-s/m]
if y0<0
   Fy = (-KG*y0)-(BG*y0);
else
    Fy=0;
end

== matlab function model1/SYSTEM/MATLAB Function ==
  data: w input; FK output; wd input; Chi input
function FK = fcn(w,wd,Chi)
k0=1; % [m]
KL=10^3; % [Nt/m]

KL2=10^5; % [Nt/m]
BL2=125; % [Nt-s/m]
if (k0-w+Chi)>0
   FK = KL*(k0-w+Chi);
else
    FK=KL2*(k0-w+Chi)-(BL2*wd);
end

== matlab function model1/SYSTEM/Control Torque ==
  data: theta1 input; theta1_d input; y0 input; tau output; theta1_des input
function tau = fcn(theta1,theta1_d,y0, theta1_des)

if y0<=0
    Kp=1800; %[Nt-m/rad]
    Kv=200; %[Nt-m-s/rad]
else
    Kp=1200; %[Nt-m/rad]
    Kv=60; %[Nt-m-s/rad]
end
tau=Kp*(theta1-theta1_des)+Kv*(theta1_d);

== matlab function model1/FILTERING AND RECONSTRUCTION/RECONSTRUCTION BLOCK/RECONSTRUCTION FUNCTION ==
  data: y2 input; w input; theta1 input; y0_r output; theta2 input
function y0_r = recontruct_y0(y2,w,theta1,theta2)
% this function reconstruct y0 from y2,theta2,theta1, values appliying
% a rounding and a FIXED SCALING

r1 = 0.5;
r2 = 0.4;

% we've to figure out an adaptive gain
gain = 0.16;


yh_temp = y2 - r2*sin(pi/2 - theta2);
y1_temp = yh_temp - (round(w) - r1).*sin(pi/2 - theta1);
y0_r = y1_temp - r1*sin(pi/2 - theta1);

if y0_r<0 
    y0_r = gain*y0_r;
end
end

== matlab function model1/FILTERING AND RECONSTRUCTION/mean ==
  data: recon input; y output; filtered input
function y = mean(recon,filtered)
% here i'm making a mean value between filtered and recon one
% i'm giving more weight to recon values

y = recon;
if recon <0
    y = 0.5*(recon+1.2*filtered);
end
